simulink model "stateflow_ex1"  (R2022a)
settings: Solver=VariableStepAuto  StartTime=0.0  StopTime=10.0  RelTol=1e-3
settings Model: PacingRate=0.100000  Creator=ArriGE66  LastModifiedBy=ArriGE66

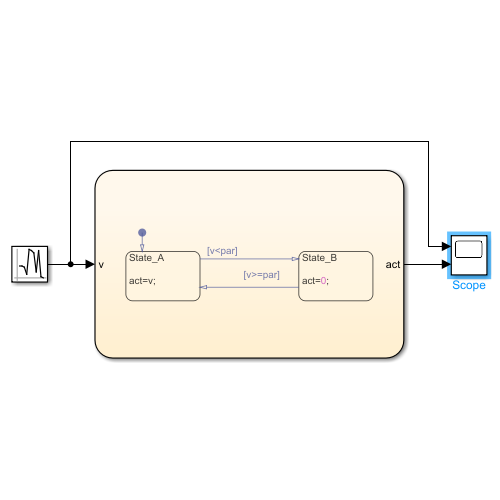
[thumbnail: Simulink's stored preview of the top-level diagram]
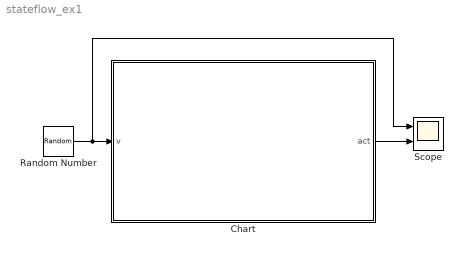
== system stateflow_ex1 ==
  Chart : Stateflow chart  TreatAsAtomicUnit=on
  Random Number : RandomNumber  SampleTime=0.1
  Scope : Scope  NumInputPorts=2
  wires:
  Random Number/1 -> Scope/1, Chart/1(v)
  Chart/1(act) -> Scope/2

== stateflow chart stateflow_ex1/Chart ==
  state State_A
    act=v;
  state State_B
    act=0;
  (default) -> State_A
  State_A -> State_B : [v<par]
  State_B -> State_A : [v>=par]
  data: act output; v input; par constant double =0
